simulink model "ACC_Project_Comfort"  (R2024b)
settings: Solver=ode4  StartTime=0.0  StopTime=60.0  FixedStep=Ts  RelTol=1e-3
values from neighbouring files (symbols this model uses):
  a_emergency = -6.0    (= -6)    [init_ACC.m]
  a_follow_min = -3.0    (= -3)    [init_ACC.m]
  a_max = 2.0    (= 2)    [init_ACC.m]    (also in matlab.mat)
  alpha_act = exp(-Ts / tau_act)    [init_ACC.m]
  d0 = 10    [init_ACC.m]    (also in matlab.mat)
  d_emergency = 45    [init_ACC.m]
  follow_off_margin = 12    [init_ACC.m]
  follow_on_margin = 5    [init_ACC.m]
  jerk_down = -3.0    (= -3)    [init_ACC.m]
  jerk_up = 1.5    [init_ACC.m]
  Kd_d = 0.8    [init_ACC.m]    (also in matlab.mat)
  Ki_v = 0    [init_ACC.m]    (also in matlab.mat = 0.08)
  Kp_d = 0.25    [init_ACC.m]    (also in matlab.mat)
  Kp_v = 0.6    [init_ACC.m]    (also in matlab.mat)
  T_gap = 1.5    [init_ACC.m]    (also in matlab.mat)
  TTC_emergency = 4.5    [init_ACC.m]
  TTC_release = 5.0    (= 5)    [init_ACC.m]
  v_ego0 = 22    [init_ACC.m]    (also in matlab.mat = 20)
  v_set = 22    [init_ACC.m]    (also in matlab.mat = 25)
  x_ego0 = 0    [init_ACC.m]    (also in matlab.mat)
  x_lead0 = 70    [init_ACC.m]    (also in matlab.mat = 60)
libraries: slpidlib x1
settings Model: Creator=jun_mac  LastModifiedBy=jun_mac

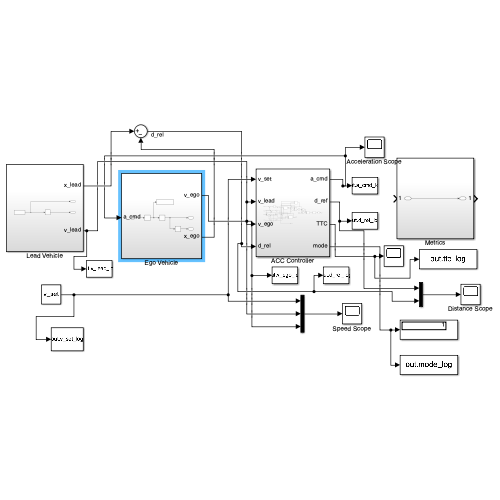
[thumbnail: Simulink's stored preview of the top-level diagram]
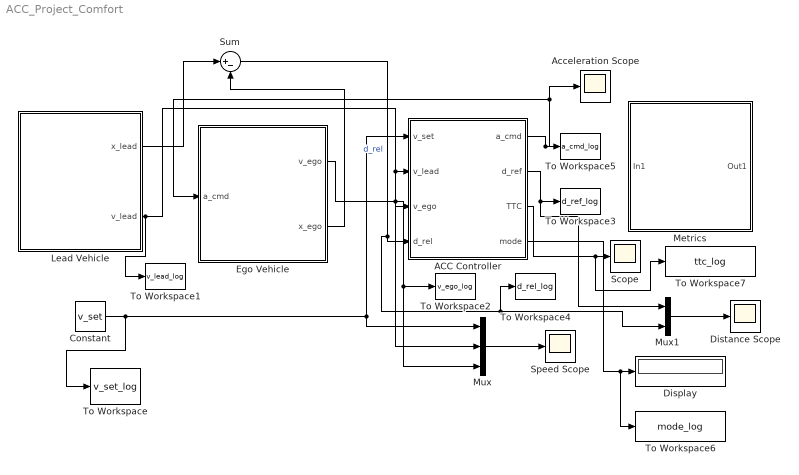
== system ACC_Project_Comfort ==
  ACC Controller : Subsystem
  Acceleration Scope : Scope
  Constant : Constant  Value=v_set
  Display : Display
  Distance Scope : Scope
  Ego Vehicle : Subsystem
  Lead Vehicle : Subsystem
  Metrics : Subsystem
  Mux : Mux  Inputs=3
  Mux1 : Mux  Inputs=2
  Scope : Scope
  Speed Scope : Scope
  Sum : Sum  Inputs=|+-
  To Workspace : ToWorkspace  VariableName=v_set_log  SaveFormat=Timeseries  SampleTime=-1
  To Workspace1 : ToWorkspace  VariableName=v_lead_log  SaveFormat=Timeseries  SampleTime=-1
  To Workspace2 : ToWorkspace  VariableName=v_ego_log  SaveFormat=Timeseries  SampleTime=-1
  To Workspace3 : ToWorkspace  VariableName=d_ref_log  SaveFormat=Timeseries  SampleTime=-1
  To Workspace4 : ToWorkspace  VariableName=d_rel_log  SaveFormat=Timeseries  SampleTime=-1
  To Workspace5 : ToWorkspace  VariableName=a_cmd_log  SaveFormat=Timeseries  SampleTime=-1
  To Workspace6 : ToWorkspace  VariableName=mode_log  SaveFormat=Timeseries  SampleTime=-1
  To Workspace7 : ToWorkspace  VariableName=ttc_log  SaveFormat=Timeseries  SampleTime=-1
  wires:
  Lead Vehicle/1(x_lead) -> Sum/1
  Ego Vehicle/2(x_ego) -> Sum/2
  Sum/1 -> To Workspace4/1, Mux1/2, ACC Controller/4(d_rel)  "d_rel"
  Ego Vehicle/1(v_ego) -> Mux/3, To Workspace2/1, ACC Controller/3(v_ego)
  Lead Vehicle/2(v_lead) -> To Workspace1/1, Mux/2, ACC Controller/2(v_lead)
  ACC Controller/1(a_cmd) -> Acceleration Scope/1, Ego Vehicle/1(a_cmd), To Workspace5/1
  Constant/1 -> To Workspace/1, Mux/1, ACC Controller/1(v_set)
  Mux/1 -> Speed Scope/1
  Mux1/1 -> Distance Scope/1
  ACC Controller/2(d_ref) -> Mux1/1, To Workspace3/1
  ACC Controller/3(TTC) -> To Workspace7/1, Scope/1
  ACC Controller/4(mode) -> To Workspace6/1, Display/1

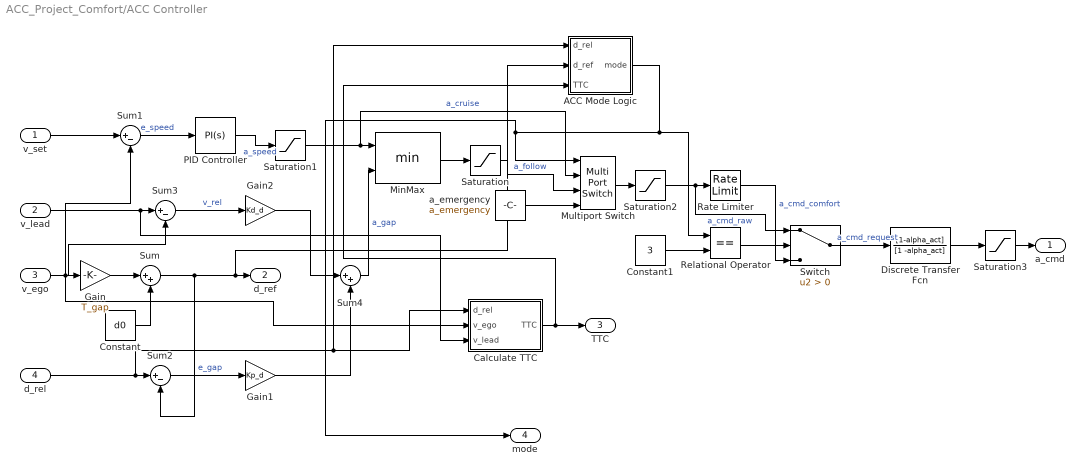
== system ACC_Project_Comfort/ACC Controller ==
  v_set : Inport
  v_lead : Inport  Port=2
  v_ego : Inport  Port=3
  d_rel : Inport  Port=4
  ACC Mode Logic : Stateflow chart  TreatAsAtomicUnit=on
  Calculate TTC : MATLAB Function  TreatAsAtomicUnit=on
  Constant : Constant  Value=d0
  Constant1 : Constant  Value=3
  Discrete Transfer Fcn : DiscreteTransferFcn  Numerator=[1-alpha_act]  Denominator=[1 -alpha_act]
  Gain : Gain  Gain=T_gap
  Gain1 : Gain  Gain=Kp_d
  Gain2 : Gain  Gain=Kd_d
  MinMax : MinMax  Inputs=2
  Multiport Switch : MultiPortSwitch  SaturateOnIntegerOverflow=off  InputSameDT=off
  PID Controller : slpidlib/PID Controller  Controller=PI  Form=Parallel  TimeDomain=Continuous-time  UseExternalTs=off  SampleTime=-1  IntegratorMethod=Forward Euler  FilterMethod=Forward Euler  ControllerParametersSource=internal  P=Kp_v  I=Ki_v  UseKiTs=off  D=0  UseExternalDerivativeSource=off  N=100  UseFilter=on  TunerSelectOption=Transfer Function Based (PID Tuner App)  InitialConditionSource=internal  InitialConditionForIntegrator=0  InitialConditionForFilter=0  DifferentiatorICPrevScaledInput=0  ExternalReset=none  TrackingMode=off  Kt=1  LimitOutput=off  SatLimitsSource=internal  UpperSaturationLimit=inf  LowerSaturationLimit=-inf  LinearizeAsGain=on  AntiWindupMode=none  Kb=1  LimitIntegrator=off  UpperIntegratorSaturationLimit=inf  LowerIntegratorSaturationLimit=-inf  POutMin=[]  POutMax=[]  IOutMin=[]  IOutMax=[]  DOutMin=[]  DOutMax=[]  NOutMin=[]  NOutMax=[]  SumOutMin=[]  SumOutMax=[]  SaturationOutMin=[]  SaturationOutMax=[]  PParamMin=[]  PParamMax=[]  IParamMin=[]  IParamMax=[]  DParamMin=[]  DParamMax=[]  NParamMin=[]  NParamMax=[]  KbParamMin=[]  KbParamMax=[]  KtParamMin=[]  KtParamMax=[]  KbOutMin=[]  KbOutMax=[]  KtOutMin=[]  KtOutMax=[]  IntegratorOutMin=[]  IntegratorOutMax=[]  FilterOutMin=[]  FilterOutMax=[]  SumI1OutMin=[]  SumI1OutMax=[]  SumI2OutMin=[]  SumI2OutMax=[]  SumI3OutMin=[]  SumI3OutMax=[]  SumI4OutMin=[]  SumI4OutMax=[]  SumDOutMin=[]  SumDOutMax=[]  DifferentiatorOutMin=[]  DifferentiatorOutMax=[]  FilterDiffOutCoefMin=[]  FilterDiffOutCoefMax=[]  ReciprocalOutMin=[]  ReciprocalOutMax=[]  SumDenOutMin=[]  SumDenOutMax=[]  SumNumOutMin=[]  SumNumOutMax=[]  DivideOutMin=[]  DivideOutMax=[]  UdiffTsProdOutMin=[]  UdiffTsProdOutMax=[]  NTsProdOutMin=[]  NTsProdOutMax=[]  UintegralTsProdOutMin=[]  UintegralTsProdOutMax=[]  UngainTsProdOutMin=[]  UngainTsProdOutMax=[]  ClampingZeroOutDataTypeStr=Inherit: Inherit via back propagation  ClampingZeroOutMin=[]  ClampingZeroOutMax=[]  FilterDenConstantOutDataTypeStr=Inherit: Inherit via back propagation  FilterDenConstantOutMin=[]  FilterDenConstantOutMax=[]  PCopyOutDataTypeStr=Inherit: Inherit via back propagation  PCopyOutMin=[]  PCopyOutMax=[]  NCopyOutDataTypeStr=Inherit: Inherit via back propagation  NCopyOutMin=[]  NCopyOutMax=[]  IntegratorContinuousStateAttributes=''  IntegratorStateMustResolveToSignalObject=off  IntegratorRTWStateStorageClass=Auto  FilterContinuousStateAttributes=''  FilterStateMustResolveToSignalObject=off  FilterRTWStateStorageClass=Auto  ParallelPVariant=InternalParameters  IdealPVariant=Disabled  IVariant=InternalParameters  DVariant=Disabled  IntegratorVariant=Continuous  SatVariant=Disabled  AWVariant=Passthrough  PCopyVariant=Disabled  TRVariant=Disabled  FdbkBlocksVariant=Forward  IdealPFdbkVariant=Disabled  SatFdbkVariant=Disabled  DerivativeFilterVariant=Disabled  NVariant=Disabled  NCopyVariant=Disabled_SignalSpec  FilterICVariant=Disabled  IntegratorICVariant=InternalICs  ExternalResetVariant=Disabled  TRSumVariant=Passthrough  SumFdbkVariant=Disabled  SumVariant=Sum_PI  TsampFilterVariant=InternalTs  TsampNgainVariant=Passthrough  TsampIntegralVariant=Disabled_SignalSpec  ExternalSaturationOutDataTypeStr=Inherit: Same as second input  DerivativeSourceVariant=Disabled  PreIntVariant=InternalPreInt
  Rate Limiter : RateLimiter  RisingSlewLimit=jerk_up  FallingSlewLimit=jerk_down  SampleTimeMode=inherited
  Relational Operator : RelationalOperator  Operator===  OutDataTypeStr=boolean  RndMeth=Simplest  InputSameDT=off
  Saturation : Saturate  UpperLimit=a_max  LowerLimit=a_follow_min
  Saturation1 : Saturate  UpperLimit=a_max  LowerLimit=a_follow_min
  Saturation2 : Saturate  UpperLimit=a_max  LowerLimit=a_emergency
  Saturation3 : Saturate  UpperLimit=a_max  LowerLimit=a_emergency
  Sum : Sum  Inputs=|++
  Sum1 : Sum  Inputs=|+-
  Sum2 : Sum  Inputs=|+-
  Sum3 : Sum  Inputs=|+-
  Sum4 : Sum  Inputs=|++
  Switch : Switch  Criteria=u2 > Threshold  SaturateOnIntegerOverflow=off  InputSameDT=off
  a_emergency : Constant  Value=a_emergency
  a_cmd : Outport
  d_ref : Outport  Port=2
  TTC : Outport  Port=3
  mode : Outport  Port=4
  wires:
  v_ego/1 -> Sum1/2, Gain/1, Sum3/2, Calculate TTC/2(v_ego)
  Gain/1 -> Sum/1
  Constant/1 -> Sum/2
  Sum/1 -> Sum2/2, ACC Mode Logic/2(d_ref), d_ref/1
  v_set/1 -> Sum1/1
  Sum1/1 -> PID Controller/1  "e_speed"
  d_rel/1 -> Calculate TTC/1(d_rel), ACC Mode Logic/1(d_rel), Sum2/1
  Sum2/1 -> Gain1/1  "e_gap"
  v_lead/1 -> Calculate TTC/3(v_lead), Sum3/1
  Sum3/1 -> Gain2/1  "v_rel"
  Gain2/1 -> Sum4/1
  Gain1/1 -> Sum4/2
  Sum4/1 -> MinMax/2  "a_gap"
  MinMax/1 -> Saturation/1
  Saturation/1 -> Multiport Switch/3  "a_follow"
  PID Controller/1 -> Saturation1/1  "a_speed"
  Saturation1/1 -> Multiport Switch/2, MinMax/1  "a_cruise"
  a_emergency/1 -> Multiport Switch/4
  Multiport Switch/1 -> Saturation2/1
  Saturation2/1 -> Switch/1, Rate Limiter/1  "a_cmd_raw"
  Calculate TTC/1(TTC) -> ACC Mode Logic/3(TTC), TTC/1
  ACC Mode Logic/1(mode) -> Relational Operator/1, Multiport Switch/1, mode/1
  Rate Limiter/1 -> Switch/3  "a_cmd_comfort"
  Constant1/1 -> Relational Operator/2
  Relational Operator/1 -> Switch/2
  Switch/1 -> Discrete Transfer Fcn/1  "a_cmd_request"
  Discrete Transfer Fcn/1 -> Saturation3/1
  Saturation3/1 -> a_cmd/1

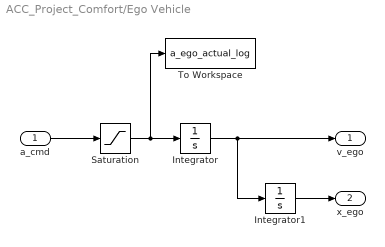
== system ACC_Project_Comfort/Ego Vehicle ==
  a_cmd : Inport
  Integrator : Integrator  InitialCondition=v_ego0  LimitOutput=on  UpperSaturationLimit=50  LowerSaturationLimit=0
  Integrator1 : Integrator  InitialCondition=x_ego0
  Saturation : Saturate  UpperLimit=a_max  LowerLimit=a_emergency
  To Workspace : ToWorkspace  VariableName=a_ego_actual_log  SaveFormat=Timeseries  SampleTime=-1
  v_ego : Outport
  x_ego : Outport  Port=2
  wires:
  a_cmd/1 -> Saturation/1
  Saturation/1 -> To Workspace/1, Integrator/1
  Integrator1/1 -> x_ego/1
  Integrator/1 -> Integrator1/1, v_ego/1

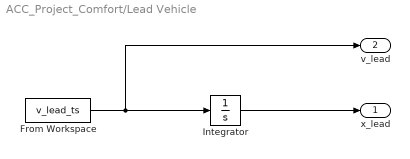
== system ACC_Project_Comfort/Lead Vehicle ==
  From Workspace : FromWorkspace  VariableName=v_lead_ts
  Integrator : Integrator  InitialCondition=x_lead0
  x_lead : Outport
  v_lead : Outport  Port=2
  wires:
  From Workspace/1 -> v_lead/1, Integrator/1
  Integrator/1 -> x_lead/1

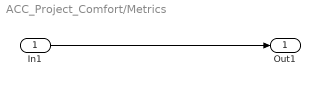
== system ACC_Project_Comfort/Metrics ==
  In1 : Inport
  Out1 : Outport
  wires:
  In1/1 -> Out1/1

== matlab function ACC_Project_Comfort/ACC Controller/Calculate TTC ==
  data: d_rel input; TTC output; v_ego input; v_lead input
function TTC = calculateTTC(d_rel, v_ego, v_lead)
%#codegen

closing_speed = v_ego - v_lead;

if d_rel <= 0
    TTC = 0;

elseif closing_speed > 0.1
    TTC = d_rel / closing_speed;

else
    TTC = 99;
end

== stateflow chart ACC_Project_Comfort/ACC Controller/ACC Mode Logic ==
  settings: updateMethod=DISCRETE  sampleTime=Ts
  state FOLLOWING
    entry:
    mode = 2;
    during:
    mode = 2;
  state CRUISE
    entry:
    mode = 1;
    during:
    mode = 1;
  state EMERGENCY
    entry:
    mode = 3;
    during:
    mode = 3;
  (default) -> CRUISE
  FOLLOWING -> CRUISE [order 2] : [d_rel >= d_ref + follow_off_margin]
  CRUISE -> EMERGENCY [order 1] : [d_rel <= d_emergency || TTC <= TTC_emergency]
  CRUISE -> FOLLOWING [order 2] : [d_rel <= d_ref + follow_on_margin]
  EMERGENCY -> FOLLOWING : [d_rel >= d_ref + 3 && TTC >= TTC_release]
  FOLLOWING -> EMERGENCY [order 1] : [d_rel <= d_emergency || TTC <= TTC_emergency]
  data: d_rel input; d_ref input; TTC input; mode output; follow_on_margin parameter; follow_off_margin parameter; d_emergency parameter; TTC_emergency parameter; TTC_release parameter
